simulink model "electric_vehicle"  (R2021a)
settings: Solver=VariableStepAuto  StartTime=0  StopTime=drive_time  RelTol=1e-3
values from neighbouring files (symbols this model uses):
  A = 2.27    [electric_vehicle_edit.m]
  bat_capacity = 36*36*(10^5)    (= 129600000)    [electric_vehicle_edit.m]
  bat_eff = 0.92    [electric_vehicle_edit.m]
  cd = 0.28    [electric_vehicle_edit.m]
  f = 0.01    [electric_vehicle_edit.m]
  g = 9.81    [electric_vehicle_edit.m]
  m = 1500    [electric_vehicle_edit.m]
  me = 1.02*m    (= 1530)    [electric_vehicle_edit.m]
  p_aksesuar = 4000    [electric_vehicle_edit.m]
  r_int = 0.1    [electric_vehicle_edit.m]
  ro_air = 1.2    [electric_vehicle_edit.m]
  rw = 0.32    [electric_vehicle_edit.m]
  transmission = 7.524    [electric_vehicle_edit.m]
  v_ocv = 350    [electric_vehicle_edit.m]
undefined symbols (not defined in the file or in its folder): eff_map, h, km, s, sigbuilder_block
libraries: simulink x4, aerolibconvert2 x2, autolibshared x1, pid_lib x1
settings Model: Creator=EKizkin  LastModifiedBy=EKizkin

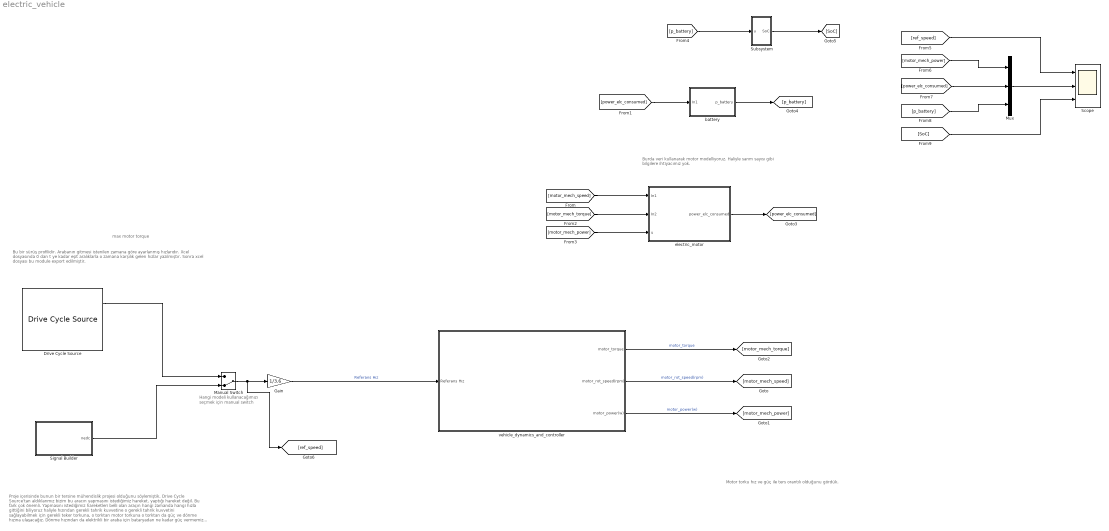
== system electric_vehicle ==
  note: Burda veri kullanarak motor modelliyoruz. Haliyle sarım sayısı gibi
      | bilgilere ihtiyacımız yok.
  note: Motor torku hız ve güç ile ters orantılı olduğunu gördük.
  note: Proje içerisinde bunun bir tersine mühendislik projesi olduğunu söylemiştik. Drive Cycle Source'tan aldıklarımız bizim bu aracın yapmasını istediğimiz hareket, yaptığı hareket değil. Bu fark çok önemli.
      |
      | Yapmasını istediğimiz hareketleri belli olan araçın hangi zamanda hangi hızla gittiğini biliyoruz haliyle hızından gerekli tahrik kuvvetine o gerekli tahrik kuvvetini sağlayabilmek için gerekli teker torkuna, o torktan  motor torkuna o torktan da güç ve dönme hızına ulaşacağız. Dönme hızından da elektrikli bir araba için bataryadan ne kadar güç vermemiz gerektiğine ulaşacağız.
  note: max motor torque
  note: Hangi modeli kullanacağımızı
      | seçmek için manual switch
  note: Bu bir sürüş profilidir. Arabanın gitmesi istenilen zamana göre ayarlanmış hızlarıdır.
      | Xcel dosyasında 0 dan t ye kadar eşit aralıklarla o zamana karşılık gelen hızlar yazılmıştır. Sonra xcel dosyası bu module export edilmiştir.
  Drive Cycle Source : autolibshared/Drive Cycle Source  cycleVar=.mat, .xls, .xlsx or .txt file  fileVar=C:\Users\EKizkin\Downloads\Project2_Electric_Vehicle\Project2_Electric_Vehicle\drive_cycle_and_effmap\wltp.xlsx  tfinal="1800  seconds"  cycleRepeat=off  outAccPort=on  outGearPort=off  gearList=No gear data  t_wot1=5  xdot_woto=0  xdot_wot1=30  t_wot2=20  xdot_wot2=0  t_wotend=30  srcUnit=km/h  outUnit=km/h  srcAccUnit=km/h/s  outAccUnit=m/s^2  dt=0  aMode=1  faultOption=off  velBnd=2  velBndUnit=mph  inUnit=m/s  timeBnd=1  failOption=off  stopSim=off  maxFaultCnt=10  maxFaultTime=2  maxTotFaultTime=15  traceOption=off  dtTrace=1  traceWindow=10  lastDCname=Custom Data Set  lastOutUnit=mph  lastDT=0  lastTB=1  lastSB=2  forceCalcBound=off
      settings: SourceProductBaseCode=PW,DR,MT,UV,VE
  Gain : Gain  Gain=1/3.6
  Manual Switch : ManualSwitch  CurrentSetting=0
  Mux : Mux  Inputs=3
  Scope : Scope  NumInputPorts=3
  Signal Builder : Subsystem  Tag=STV Subsys  LoadFcn=sigbuilder_block('load');  StartFcn=sigbuilder_block('start');  StopFcn=sigbuilder_block('stop');  ClipboardFcn=sigbuilder_block('clipboard');  mask(Sigbuilder block){tuvar=[0:10]}
      mask help: Simulink:masks:SigbuilderBlock_MD
      mask init:
      | if ~strcmp(get_param(bdroot(gcbh),'SimulationStatus'),'stopped') tuvar = sigbuilder_block('maskInit'); end
      settings: CopyFcn=sigbuilder_block('copy');  DeleteFcn=sigbuilder_block('delete');  ModelCloseFcn=sigbuilder_block('modelClose');  PreSaveFcn=sigbuilder_block('preSave');  PauseFcn=sigbuilder_block('pause');  ContinueFcn=sigbuilder_block('continue');  NameChangeFcn=sigbuilder_block('namechange');  OpenFcn=sigbuilder_block('open',[236.291 374.4 549.818 399.927 ]);  CloseFcn=sigbuilder_block('close');
      mask Display: plot(0, 0, 100, 100,[2, 2, 32, 32, 2], [68, 8, 8, 68, 68],[32, 2], [38, 38], [32, 19, 2],[53, 60, 44], [32, 17, 17, 2],[16, 16, 31, 31]);txt = getActiveGroup(gcbh);text(2, 100, txt,'verticalAlignment', 'top');
  Subsystem : Subsystem
      mask Display: image('C:\Users\EKizkin\Downloads\Project2_Electric_Vehicle\Project2_Electric_Vehicle\görsel\Measuring_Your_State_Of_Charge.jpg'); % Use "Edit Image" on toolstrip to change.
  battery : Subsystem
      mask Display: image('C:\Users\EKizkin\Downloads\Project2_Electric_Vehicle\Project2_Electric_Vehicle\görsel\Screenshot (411).png'); % Use "Edit Image" on toolstrip to change.
  electric_motor : Subsystem
      mask Display: image('C:\Users\EKizkin\Downloads\Project2_Electric_Vehicle\Project2_Electric_Vehicle\görsel\DC-motor-parts.png'); % Use "Edit Image" on toolstrip to change.
  vehicle_dynamics_and_controller : Subsystem
      mask Display: image('C:\Users\EKizkin\Downloads\Project2_Electric_Vehicle\Project2_Electric_Vehicle\görsel\Nissan_Leaf_2018-17.jpg'); % Use "Edit Image" on toolstrip to change.
  wires:
  Drive Cycle Source/1 -> Manual Switch/1
  Signal Builder/1(nedc) -> Manual Switch/2
  Manual Switch/1 -> [ref_speed], Gain/1
  Gain/1 -> vehicle_dynamics_and_controller/1(Referans Hız)  "Referans Hız"
  vehicle_dynamics_and_controller/1(motor_torque) -> [motor_mech_torque]  "motor_torque"
  vehicle_dynamics_and_controller/2(motor_rot_speed(rpm)) -> [motor_mech_speed]  "motor_rot_speed(rpm)"
  vehicle_dynamics_and_controller/3(motor_power(w)) -> [motor_mech_power]  "motor_power(w)"
  [motor_mech_speed] -> electric_motor/1(In1)
  [motor_mech_torque] -> electric_motor/2(In2)
  [motor_mech_power] -> electric_motor/3(u)
  electric_motor/1(power_elc_consumed) -> [power_elc_consumed]
  [power_elc_consumed] -> battery/1(In1)
  battery/1(p_battery) -> [p_battery]
  [p_battery] -> Subsystem/1(u)
  Subsystem/1(SoC) -> [SoC]
  [motor_mech_power] -> Mux/1
  [power_elc_consumed] -> Mux/2
  [p_battery] -> Mux/3
  Mux/1 -> Scope/2
  [ref_speed] -> Scope/1
  [SoC] -> Scope/3

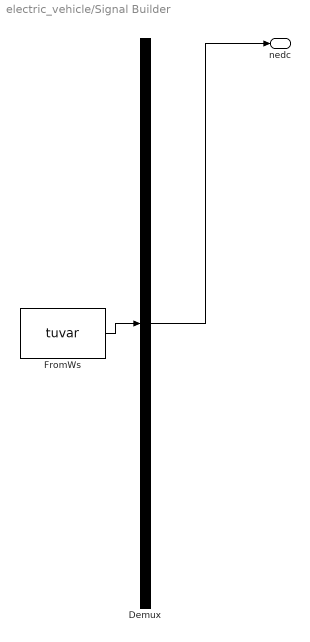
== system electric_vehicle/Signal Builder ==
  Demux : Demux  Tag=STV Demux  Outputs=1
      settings: DisplayOption=none
  FromWs : FromWorkspace  Tag=STV FromWs  VariableName=tuvar
      SigBuilderData=|
      | common.afterFinalStr = 'Extrapolate'
      | common.sampleTime = 0
      | dataSet.timeRange = [0 1180]
      | dataSet.name = 'Group 1'
      | sbobj.Groups.Name = 'Group 1'
      | sbobj.Groups.Signals.Name = 'nedc'
      | sbobj.Groups.Signals.XData = [0 2 3 4 5 6 7 8 9 10 11 12 ... (1180 elements, 1x1180)]
      | sbobj.Groups.Signals.YData = [0 0 0 0 0 0 0 0 0 0 0 3.8 ... (1180 elements, 1x1180)]
      | sbobj.Groups.TimeRange = [0 1180]
  nedc : Outport  Tag=STV Outport
  wires:
  Demux/1 -> nedc/1
  FromWs/1 -> Demux/1

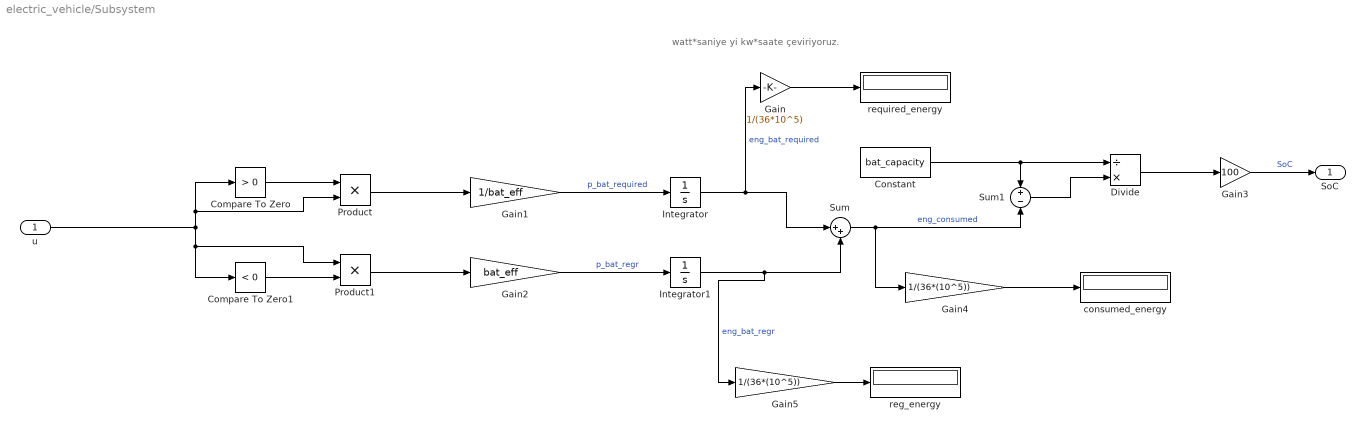
== system electric_vehicle/Subsystem ==
  note: watt*saniye yi kw*saate çeviriyoruz.
  u : Inport
  Compare To Zero : simulink/Logic and Bit Operations/Compare To Zero  relop=>  OutDataTypeStr=boolean
  Compare To Zero1 : simulink/Logic and Bit Operations/Compare To Zero  relop=<  OutDataTypeStr=boolean
  Constant : Constant  Value=bat_capacity
  Divide : Product  Inputs=/*
  Gain : Gain  Gain=1/(36*10^5)
  Gain1 : Gain  Gain=1/bat_eff
  Gain2 : Gain  Gain=bat_eff
  Gain3 : Gain  Gain=100
  Gain4 : Gain  Gain=1/(36*(10^5))
  Gain5 : Gain  Gain=1/(36*(10^5))
  Integrator : Integrator
  Integrator1 : Integrator
  Product : Product
  Product1 : Product
  Sum : Sum  Inputs=|++
  Sum1 : Sum  Inputs=+-
  consumed_energy : Display
  reg_energy : Display
  required_energy : Display
  SoC : Outport
  wires:
  Gain2/1 -> Integrator1/1  "p_bat_regr"
  u/1 -> Product1/1, Compare To Zero1/1, Product/2, Compare To Zero/1
  Divide/1 -> Gain3/1
  Sum1/1 -> Divide/2
  Product/1 -> Gain1/1
  Gain3/1 -> SoC/1  "SoC"
  Gain1/1 -> Integrator/1  "p_bat_required"
  Product1/1 -> Gain2/1
  Compare To Zero1/1 -> Product1/2
  Sum/1 -> Gain4/1, Sum1/2  "eng_consumed"
  Integrator/1 -> Gain/1, Sum/1  "eng_bat_required"
  Integrator1/1 -> Gain5/1, Sum/2  "eng_bat_regr"
  Constant/1 -> Sum1/1, Divide/1
  Compare To Zero/1 -> Product/1
  Gain/1 -> required_energy/1
  Gain5/1 -> reg_energy/1
  Gain4/1 -> consumed_energy/1

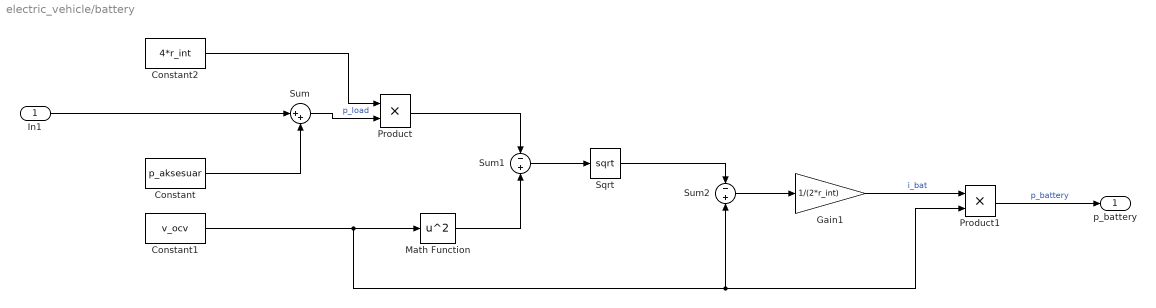
== system electric_vehicle/battery ==
  In1 : Inport
  Constant : Constant  Value=p_aksesuar
  Constant1 : Constant  Value=v_ocv
  Constant2 : Constant  Value=4*r_int
  Gain1 : Gain  Gain=1/(2*r_int)
  Math Function : Math  Operator=square  SaturateOnIntegerOverflow=on
  Product : Product
  Product1 : Product
  Sqrt : Sqrt  SaturateOnIntegerOverflow=on
  Sum : Sum  Inputs=|++
  Sum1 : Sum  Inputs=-+
  Sum2 : Sum  Inputs=-+
  p_battery : Outport
  wires:
  Sqrt/1 -> Sum2/1
  Gain1/1 -> Product1/1  "i_bat"
  Constant/1 -> Sum/2
  Constant1/1 -> Math Function/1, Product1/2, Sum2/2
  Math Function/1 -> Sum1/2
  Sum/1 -> Product/2  "p_load"
  Product/1 -> Sum1/1
  Sum2/1 -> Gain1/1
  Sum1/1 -> Sqrt/1
  Constant2/1 -> Product/1
  In1/1 -> Sum/1
  Product1/1 -> p_battery/1  "p_battery"

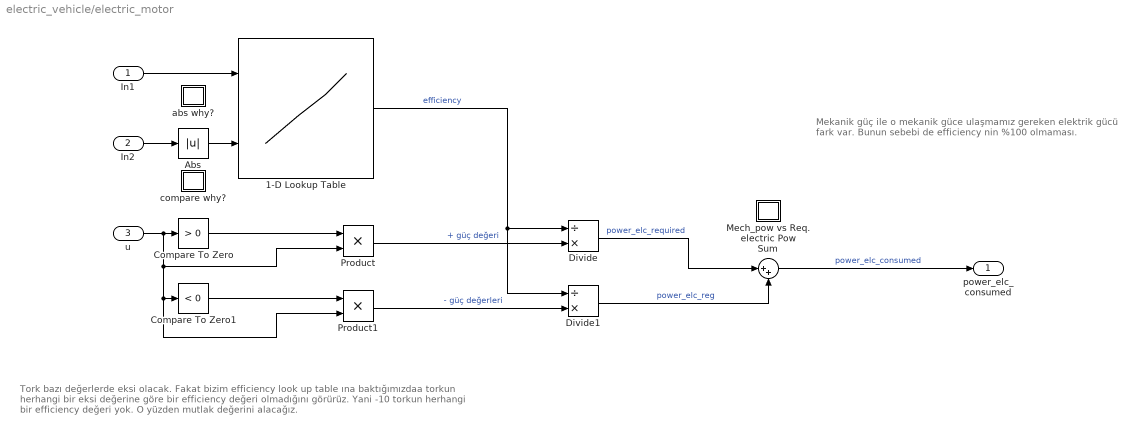
== system electric_vehicle/electric_motor ==
  note: Mekanik güç ile o mekanik güce ulaşmamız gereken elektrik gücü fark var.
      | Bunun sebebi de efficiency nin %100 olmaması.
  note: Tork bazı değerlerde eksi olacak. Fakat bizim efficiency look up table ına baktığımızdaa
      | torkun herhangi bir eksi değerine göre bir efficiency değeri olmadığını görürüz. Yani -10 torkun herhangi bir efficiency değeri yok. O yüzden mutlak değerini alacağız.
  In1 : Inport
  In2 : Inport  Port=2
  u : Inport  Port=3
  1-D Lookup Table : Lookup_n-D  BreakpointsForDimension1=eff_map.speed  BreakpointsForDimension2=eff_map.torque  Table=eff_map.efficiency  InternalRulePriority=Speed  RndMeth=Simplest  InputSameDT=on
      settings: InputPortMap=u0,u1
  Abs : Abs
  Compare To Zero : simulink/Logic and Bit Operations/Compare To Zero  relop=>  OutDataTypeStr=boolean
  Compare To Zero1 : simulink/Logic and Bit Operations/Compare To Zero  relop=<  OutDataTypeStr=boolean
  Divide : Product  Inputs=/*
  Divide1 : Product  Inputs=/*
  Mech_pow vs Req. electric Pow : Stateflow chart  TreatAsAtomicUnit=on
  Product : Product
  Product1 : Product
  Sum : Sum  Inputs=|++
  abs why? : Stateflow chart  TreatAsAtomicUnit=on
  compare why? : Stateflow chart  TreatAsAtomicUnit=on
  power_elc_consumed : Outport
  wires:
  Divide/1 -> Sum/1  "power_elc_required"
  1-D Lookup Table/1 -> Divide1/1, Divide/1  "efficiency"
  Abs/1 -> 1-D Lookup Table/2
  Product1/1 -> Divide1/2  "- güç değerleri"
  In1/1 -> 1-D Lookup Table/1
  Compare To Zero/1 -> Product/1
  u/1 -> Product/2, Product1/2, Compare To Zero1/1, Compare To Zero/1
  Divide1/1 -> Sum/2  "power_elc_reg"
  Compare To Zero1/1 -> Product1/1
  Product/1 -> Divide/2  "+ güç değeri"
  Sum/1 -> power_elc_consumed/1  "power_elc_consumed"
  In2/1 -> Abs/1

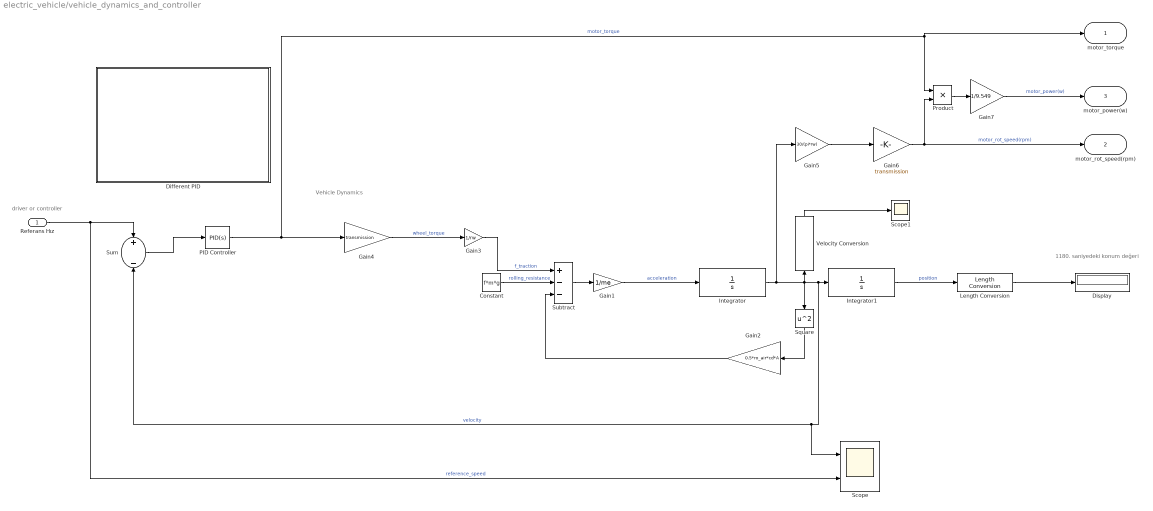
== system electric_vehicle/vehicle_dynamics_and_controller ==
  note: driver or controller
  note: Vehicle Dynamics
  note: 1180. saniyedeki konum değeri
  Referans Hız : Inport
  Constant : Constant  Value=f*m*g
  Different PID : Stateflow chart  TreatAsAtomicUnit=on
  Display : Display
  Gain1 : Gain  Gain=1/me
  Gain2 : Gain  Gain=0.5*ro_air*cd*A
  Gain3 : Gain  Gain=1/rw
  Gain4 : Gain  Gain=transmission
  Gain5 : Gain  Gain=30/(pi*rw)
  Gain6 : Gain  Gain=transmission
  Gain7 : Gain  Gain=1/9.549
  Integrator : Integrator
  Integrator1 : Integrator
  Length Conversion : aerolibconvert2/Length Conversion  IU=m  OU=km
  PID Controller : pid_lib/PID Controller  Controller=PID  Form=Parallel  TimeDomain=Continuous-time  UseExternalTs=off  SampleTime=-1  IntegratorMethod=Forward Euler  FilterMethod=Forward Euler  ControllerParametersSource=internal  P=620.656823334484  I=1096.26740706283  D=11.7869770659031  UseFilter=on  N=36.46824066771  TunerSelectOption=Transfer Function Based (PID Tuner App)  InitialConditionSource=internal  InitialConditionForIntegrator=0  InitialConditionForFilter=0  DifferentiatorICPrevScaledInput=0  ExternalReset=none  TrackingMode=off  Kt=1  LimitOutput=off  SatLimitsSource=internal  UpperSaturationLimit=inf  LowerSaturationLimit=-inf  LinearizeAsGain=on  AntiWindupMode=none  Kb=1  POutMin=[]  POutMax=[]  IOutMin=[]  IOutMax=[]  DOutMin=[]  DOutMax=[]  NOutMin=[]  NOutMax=[]  SumOutMin=[]  SumOutMax=[]  SaturationOutMin=[]  SaturationOutMax=[]  PParamMin=[]  PParamMax=[]  IParamMin=[]  IParamMax=[]  DParamMin=[]  DParamMax=[]  NParamMin=[]  NParamMax=[]  KbParamMin=[]  KbParamMax=[]  KtParamMin=[]  KtParamMax=[]  KbOutMin=[]  KbOutMax=[]  KtOutMin=[]  KtOutMax=[]  IntegratorOutMin=[]  IntegratorOutMax=[]  FilterOutMin=[]  FilterOutMax=[]  SumI1OutMin=[]  SumI1OutMax=[]  SumI2OutMin=[]  SumI2OutMax=[]  SumI3OutMin=[]  SumI3OutMax=[]  SumI4OutMin=[]  SumI4OutMax=[]  SumDOutMin=[]  SumDOutMax=[]  DifferentiatorOutMin=[]  DifferentiatorOutMax=[]  FilterDiffOutCoefMin=[]  FilterDiffOutCoefMax=[]  ReciprocalOutMin=[]  ReciprocalOutMax=[]  SumDenOutMin=[]  SumDenOutMax=[]  SumNumOutMin=[]  SumNumOutMax=[]  DivideOutMin=[]  DivideOutMax=[]  UdiffTsProdOutMin=[]  UdiffTsProdOutMax=[]  NTsProdOutMin=[]  NTsProdOutMax=[]  UintegralTsProdOutMin=[]  UintegralTsProdOutMax=[]  UngainTsProdOutMin=[]  UngainTsProdOutMax=[]  IntegratorContinuousStateAttributes=''  IntegratorStateMustResolveToSignalObject=off  IntegratorRTWStateStorageClass=Auto  FilterContinuousStateAttributes=''  FilterStateMustResolveToSignalObject=off  FilterRTWStateStorageClass=Auto  ParallelPVariant=InternalParameters  IdealPVariant=Disabled  IVariant=InternalParameters  DVariant=InternalParameters  IntegratorVariant=Continuous  SatVariant=Disabled  AWVariant=Passthrough  PCopyVariant=Disabled  TRVariant=Disabled  FdbkBlocksVariant=Forward  IdealPFdbkVariant=Disabled  SatFdbkVariant=Disabled  DerivativeFilterVariant=ContFilter  NVariant=InternalParameters  NCopyVariant=Disabled  FilterICVariant=InternalICsFilter  IntegratorICVariant=InternalICs  ExternalResetVariant=Disabled  TRSumVariant=Passthrough  SumFdbkVariant=Disabled  SumVariant=Sum_PID  TsampFilterVariant=InternalTs  TsampNgainVariant=Passthrough  TsampIntegralVariant=Passthrough  ExternalSaturationOutDataTypeStr=Inherit: Same as second input
  Product : Product
  Scope : Scope  NumInputPorts=2
  Scope1 : Scope
  Square : Math  Operator=square  SaturateOnIntegerOverflow=on
  Subtract : Sum  Inputs=+--
  Sum : Sum  Inputs=+-
  Velocity Conversion : aerolibconvert2/Velocity Conversion  IU=m/s  OU=km/h
  motor_torque : Outport
  motor_rot_speed(rpm) : Outport  Port=2
  motor_power(w) : Outport  Port=3
  wires:
  Referans Hız/1 -> Scope/2, Sum/1  "reference_speed"
  Integrator/1 -> Gain5/1, Scope/1, Sum/2, Integrator1/1, Velocity Conversion/1, Square/1  "velocity"
  PID Controller/1 -> Gain4/1, motor_torque/1, Product/1  "motor_torque"
  Gain7/1 -> motor_power(w)/1  "motor_power(w)"
  Gain4/1 -> Gain3/1  "wheel_torque"
  Gain6/1 -> motor_rot_speed(rpm)/1, Product/2  "motor_rot_speed(rpm)"
  Length Conversion/1 -> Display/1
  Square/1 -> Gain2/1
  Sum/1 -> PID Controller/1
  Subtract/1 -> Gain1/1
  Constant/1 -> Subtract/2  "rolling_resistance"
  Gain3/1 -> Subtract/1  "f_traction"
  Gain2/1 -> Subtract/3
  Gain1/1 -> Integrator/1  "acceleration"
  Product/1 -> Gain7/1
  Velocity Conversion/1 -> Scope1/1
  Integrator1/1 -> Length Conversion/1  "position"
  Gain5/1 -> Gain6/1

== stateflow chart electric_vehicle/electric_motor/abs why? ==
  note: Tork bazı değerlerde eksi olacak. Fakat bizim efficiency look up table ına baktığımızda
      | torkun herhangi bir eksi değerine göre bir efficiency değeri olmadığını görürüz.
      | Yani -10 torkun herhangi bir efficiency değeri yok. O yüzden mutlak değerini alacağız.
  note: Birinci PID düzenimizde katsayılarımız:
      |
      | kp:63.03
      | ki:12.17
      | kd:-17.28
  note: İkinci PID düzenimizde katsayılarımız:
      |
      | kp:620.66
      | ki:1096.27
      | kd:11.79
  note: 1. fotoda istenilen(mavi) ve gerçekleşen arasındaki fark ile 2. fotoda istenilen ve gerçekleştirilen arasındaki fark incelenebilir.

== stateflow chart electric_vehicle/electric_motor/compare why? ==
  note: Efficiency değerlerini elde ettik ama formuller gücün - ve + olduğu yerler için farklıydı. Haliyle gücü - lduğu ve + olduğu yerlerde farklı fonksiyonlara sokmamız gerekiyor.
  note: Birinci PID düzenimizde katsayılarımız:
      |
      | kp:63.03
      | ki:12.17
      | kd:-17.28
  note: İkinci PID düzenimizde katsayılarımız:
      |
      | kp:620.66
      | ki:1096.27
      | kd:11.79
  note: 1. fotoda istenilen(mavi) ve gerçekleşen arasındaki fark ile 2. fotoda istenilen ve gerçekleştirilen arasındaki fark incelenebilir.

== stateflow chart electric_vehicle/vehicle_dynamics_and_controller/Different PID ==
  note: PID'de kp,ki,kd gibi parametreler olduğunu biliyoruz. Bu parametreler bizim drive sourceta istenilen profili ne kadar keskin bir şekilde ne kadar sürede yakalayacağımızı belirliyor. Bunu daha iyi anlayabilmek için PID componentindeki tune'da iki farklı profil oluşturucam. Ve bu farklı profillerin
      | istenilen drive cycle a ne kadar yakın olduklarını ne kadar sürede bu drive cycle'ı yakaladıklarınız göreceğiz.
  note: Birinci PID düzenimizde katsayılarımız:
      |
      | kp:63.03
      | ki:12.17
      | kd:-17.28
  note: İkinci PID düzenimizde katsayılarımız:
      |
      | kp:620.66
      | ki:1096.27
      | kd:11.79
  note: ?
  note: ?
  note: 1. fotoda istenilen(mavi) ve gerçekleşen arasındaki fark ile 2. fotoda istenilen ve gerçekleştirilen arasındaki fark incelenebilir.

== stateflow chart electric_vehicle/electric_motor/Mech_pow vs Req. electric Pow ==
  note: ?
  note: Böyle bir karşılaştırma istediğimiz mekanik motor gücü ile o mekanik güce
      | ulaşmamız gereken gerekli elektrik gücünü karşılaştırmak için harika bir fırsat.
      | Harcamamız gereken gücün her zaman mekanik güçten fazla olduğuna dikkat çekilmeli.
      |  Bunun sebebi verimin (efficiency) nin yüzde yüz olmaması.
  note: ?
  note: Sarı: verilmesi gereken güç
      | Mavi: Motorun mekanik gücü
  note: Birinci PID düzenimizde katsayılarımız:
      |
      | kp:63.03
      | ki:12.17
      | kd:-17.28
  note: İkinci PID düzenimizde katsayılarımız:
      |
      | kp:620.66
      | ki:1096.27
      | kd:11.79
  note: 1. fotoda istenilen(mavi) ve gerçekleşen arasındaki fark ile 2. fotoda istenilen ve gerçekleştirilen arasındaki fark incelenebilir.
